simulink subsystem "led2023V"  (R2023b)
settings: Solver=VariableStepAuto  StartTime=0.0  StopTime=10.0  RelTol=1e-3
libraries: arduinolib x3
settings Model: Creator=Usuario_UMA  LastModifiedBy=juana

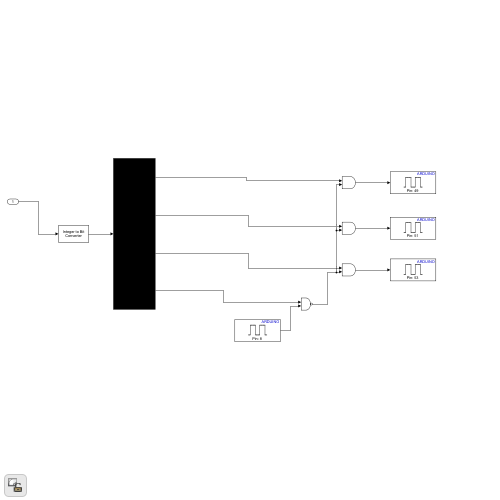
[thumbnail: Simulink's stored preview of the top-level diagram]
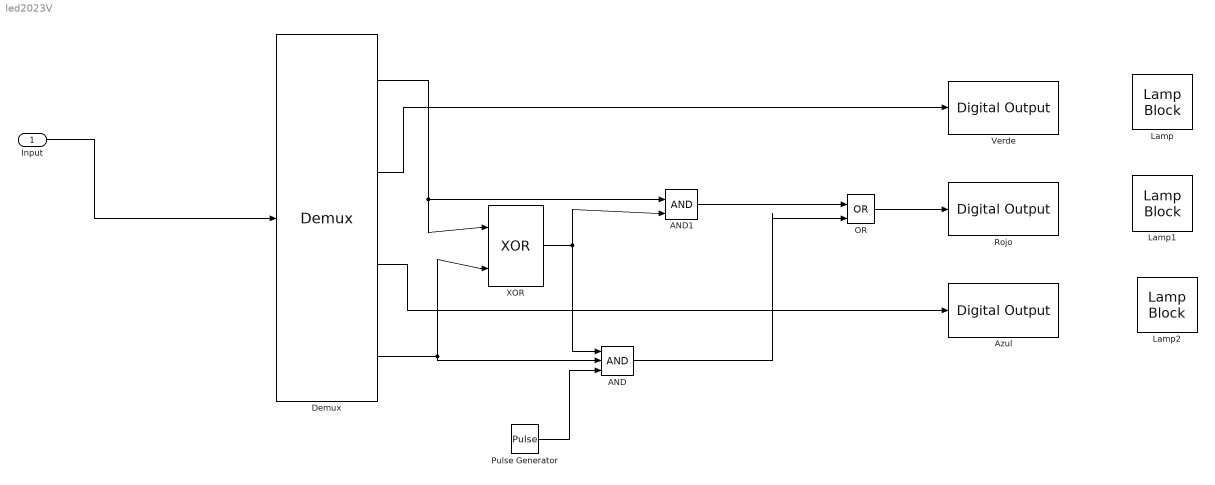
== system led2023V ==
  Input : Inport
  AND : Logic  Inputs=3  IconShape=distinctive  AllPortsSameDT=off  OutDataTypeStr=boolean
  AND1 : Logic  IconShape=distinctive  AllPortsSameDT=off  OutDataTypeStr=boolean
  Azul : arduinolib/Digital Output  pinNumber=49  Direction=output  blockPlatform=arduino
  Demux : Demux
  Lamp : LampBlock  LabelPosition=Hide
  Lamp1 : LampBlock  LabelPosition=Hide
  Lamp2 : LampBlock  LabelPosition=Hide
  OR : Logic  Operator=OR  IconShape=distinctive  AllPortsSameDT=off  OutDataTypeStr=boolean
  Pulse Generator : DiscretePulseGenerator  PulseType=Time based  Period=1  PulseWidth=50
  Rojo : arduinolib/Digital Output  pinNumber=51  Direction=output  blockPlatform=arduino
  Verde : arduinolib/Digital Output  pinNumber=53  Direction=output  blockPlatform=arduino
  XOR : Logic  Operator=XOR  IconShape=distinctive  AllPortsSameDT=off  OutDataTypeStr=boolean
  wires:
  Input/1 -> Demux/1
  Demux/4 -> AND/2, XOR/2
  Pulse Generator/1 -> AND/3
  Demux/1 -> XOR/1, AND1/1
  XOR/1 -> AND/1, AND1/2
  OR/1 -> Rojo/1
  AND1/1 -> OR/1
  AND/1 -> OR/2
  Demux/3 -> Azul/1
  Demux/2 -> Verde/1
